simulink model "DLH_nguocslx"  (R2020a)
settings: Solver=VariableStepAuto  StartTime=0.0  StopTime=10.0  RelTol=1e-3
settings Model: Creator=dell  LastModifiedBy=dell

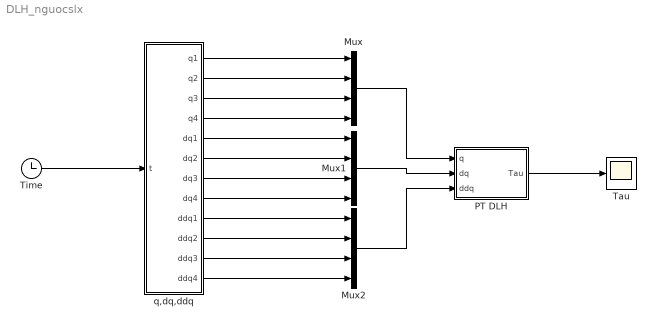
== system DLH_nguocslx ==
  Mux : Mux
  Mux1 : Mux
  Mux2 : Mux
  "PT DLH " : MATLAB Function  TreatAsAtomicUnit=on
  Tau : Scope
  Time : Clock
  q,dq,ddq : MATLAB Function  TreatAsAtomicUnit=on
  wires:
  Time/1 -> q,dq,ddq/1(t)
  q,dq,ddq/1(q1) -> Mux/1
  q,dq,ddq/2(q2) -> Mux/2
  q,dq,ddq/3(q3) -> Mux/3
  q,dq,ddq/4(q4) -> Mux/4
  q,dq,ddq/6(dq2) -> Mux1/2
  q,dq,ddq/5(dq1) -> Mux1/1
  q,dq,ddq/7(dq3) -> Mux1/3
  q,dq,ddq/8(dq4) -> Mux1/4
  q,dq,ddq/9(ddq1) -> Mux2/1
  q,dq,ddq/10(ddq2) -> Mux2/2
  q,dq,ddq/11(ddq3) -> Mux2/3
  q,dq,ddq/12(ddq4) -> Mux2/4
  Mux/1 -> "PT DLH "/1(q)
  Mux1/1 -> "PT DLH "/2(dq)
  Mux2/1 -> "PT DLH "/3(ddq)
  "PT DLH "/1(Tau) -> Tau/1

== matlab function DLH_nguocslx/PT DLH  ==
  data: q input; Tau output; dq input; ddq input
function Tau = fcn(q,dq,ddq)

[L1, L2, L3, L4,L0,m1,m2,m3,m4,I1x,I1y,I1z,I2x,I2y,I2z,I3x,I3y,I3z,I4x,I4y,I4z]=Parameters();

M=zeros(4,4);
M(1,1)= m1 + m2 + m3 + m4;
M(1,2)= ((-0.3e1 * m4 * L4 * cos(q(4)) - 0.3e1 * L3 * (m3 + 0.2e1 / 0.3e1 * m4)) * cos(q(3)) + 0.3e1 * sin(q(3)) * sin(q(4)) * L4 * m4 - 0.3e1 * L2 * (m2 + 0.2e1 / 0.3e1 * m3 + 0.2e1 / 0.3e1 * m4)) * cos(q(2)) / 0.2e1 + 0.3e1 / 0.2e1 * sin(q(2)) * (sin(q(4)) * L4 * m4 * cos(q(3)) + (m4 * L4 * cos(q(4)) + L3 * (m3 + 0.2e1 / 0.3e1 * m4)) * sin(q(3)));
M(1,3)= ((-0.3e1 * m4 * L4 * cos(q(4)) - 0.3e1 * L3 * (m3 + 0.2e1 / 0.3e1 * m4)) * cos(q(3)) + 0.3e1 * sin(q(3)) * sin(q(4)) * L4 * m4) * cos(q(2)) / 0.2e1 + 0.3e1 / 0.2e1 * sin(q(2)) * (sin(q(4)) * L4 * m4 * cos(q(3)) + (m4 * L4 * cos(q(4)) + L3 * (m3 + 0.2e1 / 0.3e1 * m4)) * sin(q(3)));
M(1,4)= 0.3e1 / 0.2e1 * L4 * ((sin(q(2)) * sin(q(3)) - cos(q(2)) * cos(q(3))) * cos(q(4)) + sin(q(4)) * (cos(q(2)) * sin(q(3)) + sin(q(2)) * cos(q(3)))) * m4;

M(2,1)= ((-0.3e1 * m4 * L4 * cos(q(4)) - 0.3e1 * L3 * (m3 + 0.2e1 / 0.3e1 * m4)) * cos(q(3)) + 0.3e1 * sin(q(3)) * sin(q(4)) * L4 * m4 - 0.3e1 * L2 * (m2 + 0.2e1 / 0.3e1 * m3 + 0.2e1 / 0.3e1 * m4)) * cos(q(2)) / 0.2e1 + 0.3e1 / 0.2e1 * sin(q(2)) * (sin(q(4)) * L4 * m4 * cos(q(3)) + (m4 * L4 * cos(q(4)) + L3 * (m3 + 0.2e1 / 0.3e1 * m4)) * sin(q(3)));
M(2,2)= 0.3e1 * L2 * (m4 * L4 * cos(q(4)) + L3 * (m3 + 0.2e1 / 0.3e1 * m4)) * cos(q(3)) + 0.3e1 * m4 * L4 * L3 * cos(q(4)) - 0.3e1 * m4 * L4 * L2 * sin(q(4)) * sin(q(3)) + ((9 * m2) + 0.4e1 * m3 + 0.4e1 * m4) * L2 ^ 2 / 0.4e1 + (0.4e1 * L3 ^ 2 + 0.9e1 * L4 ^ 2) * m4 / 0.4e1 + 0.9e1 / 0.4e1 * m3 * L3 ^ 2 + I3z + I4z + I2z;
M(2,3)= 0.3e1 / 0.2e1 * L2 * (m4 * L4 * cos(q(4)) + L3 * (m3 + 0.2e1 / 0.3e1 * m4)) * cos(q(3)) + 0.3e1 * m4 * L4 * L3 * cos(q(4)) - 0.3e1 / 0.2e1 * m4 * L4 * L2 * sin(q(4)) * sin(q(3)) + (0.4e1 * L3 ^ 2 + 0.9e1 * L4 ^ 2) * m4 / 0.4e1 + 0.9e1 / 0.4e1 * m3 * L3 ^ 2 + I3z + I4z;
M(2,4)= 0.3e1 / 0.2e1 * m4 * L4 * (L2 * cos(q(3)) + L3) * cos(q(4)) - 0.3e1 / 0.2e1 * m4 * L4 * L2 * sin(q(4)) * sin(q(3)) + 0.9e1 / 0.4e1 * m4 * L4 ^ 2 + I4z;

M(3,1)= ((-0.3e1 * m4 * L4 * cos(q(4)) - 0.3e1 * L3 * (m3 + 0.2e1 / 0.3e1 * m4)) * cos(q(3)) + 0.3e1 * sin(q(3)) * sin(q(4)) * L4 * m4) * cos(q(2)) / 0.2e1 + 0.3e1 / 0.2e1 * sin(q(2)) * (sin(q(4)) * L4 * m4 * cos(q(3)) + (m4 * L4 * cos(q(4)) + L3 * (m3 + 0.2e1 / 0.3e1 * m4)) * sin(q(3)));
M(3,2)= 0.3e1 / 0.2e1 * L2 * (m4 * L4 * cos(q(4)) + L3 * (m3 + 0.2e1 / 0.3e1 * m4)) * cos(q(3)) + 0.3e1 * m4 * L4 * L3 * cos(q(4)) - 0.3e1 / 0.2e1 * m4 * L4 * L2 * sin(q(4)) * sin(q(3)) + (0.4e1 * L3 ^ 2 + 0.9e1 * L4 ^ 2) * m4 / 0.4e1 + 0.9e1 / 0.4e1 * m3 * L3 ^ 2 + I3z + I4z;
M(3,3)= 0.3e1 * m4 * L4 * L3 * cos(q(4)) + ((9 * m3) + 0.4e1 * m4) * L3 ^ 2 / 0.4e1 + 0.9e1 / 0.4e1 * m4 * L4 ^ 2 + I3z + I4z;
M(3,4)= 0.3e1 / 0.2e1 * m4 * L4 * L3 * cos(q(4)) + 0.9e1 / 0.4e1 * m4 * L4 ^ 2 + I4z;

M(4,1)= 0.3e1 / 0.2e1 * L4 * ((sin(q(2)) * sin(q(3)) - cos(q(2)) * cos(q(3))) * cos(q(4)) + sin(q(4)) * (cos(q(2)) * sin(q(3)) + sin(q(2)) * cos(q(3)))) * m4;
M(4,2)= 0.3e1 / 0.2e1 * m4 * L4 * (L2 * cos(q(3)) + L3) * cos(q(4)) - 0.3e1 / 0.2e1 * m4 * L4 * L2 * sin(q(4)) * sin(q(3)) + 0.9e1 / 0.4e1 * m4 * L4 ^ 2 + I4z;
M(4,3)= 0.3e1 / 0.2e1 * m4 * L4 * L3 * cos(q(4)) + 0.9e1 / 0.4e1 * m4 * L4 ^ 2 + I4z;
M(4,4)= 0.9e1 / 0.4e1 * m4 * L4 ^ 2 + I4z;

C=zeros(4,4);

C(1,1)= 0;
C(1,2)= ((0.3e1 * L4 * m4 * (dq(3) + dq(4) + dq(2)) * cos(q(4)) + 0.3e1 * L3 * (dq(3) + dq(2)) * (m3 + 0.2e1 / 0.3e1 * m4)) * cos(q(3)) - 0.3e1 * sin(q(3)) * sin(q(4)) * L4 * m4 * (dq(3) + dq(4) + dq(2)) + 0.3e1 * dq(2) * L2 * (m2 + 0.2e1 / 0.3e1 * m3 + 0.2e1 / 0.3e1 * m4)) * sin(q(2)) / 0.2e1 + 0.3e1 / 0.2e1 * cos(q(2)) * (sin(q(4)) * L4 * m4 * (dq(3) + dq(4) + dq(2)) * cos(q(3)) + sin(q(3)) * (L4 * m4 * (dq(3) + dq(4) + dq(2)) * cos(q(4)) + L3 * (dq(3) + dq(2)) * (m3 + 0.2e1 / 0.3e1 * m4)));
C(1,3)= (0.3e1 * sin(q(4)) * L4 * m4 * (dq(3) + dq(4) + dq(2)) * cos(q(3)) + 0.3e1 * sin(q(3)) * (L4 * m4 * (dq(3) + dq(4) + dq(2)) * cos(q(4)) + L3 * (dq(3) + dq(2)) * (m3 + 0.2e1 / 0.3e1 * m4))) * cos(q(2)) / 0.2e1 + 0.3e1 / 0.2e1 * ((L4 * m4 * (dq(3) + dq(4) + dq(2)) * cos(q(4)) + L3 * (dq(3) + dq(2)) * (m3 + 0.2e1 / 0.3e1 * m4)) * cos(q(3)) - sin(q(3)) * sin(q(4)) * L4 * m4 * (dq(3) + dq(4) + dq(2))) * sin(q(2));
C(1,4)= 0.3e1 / 0.2e1 * L4 * ((cos(q(2)) * sin(q(3)) + sin(q(2)) * cos(q(3))) * cos(q(4)) + (cos(q(2)) * cos(q(3)) - sin(q(2)) * sin(q(3))) * sin(q(4))) * (dq(3) + dq(4) + dq(2)) * m4;

C(2,1)= ((0.3e1 * L4 * m4 * (dq(3) + dq(4) + dq(2)) * cos(q(4)) + 0.3e1 * L3 * (m3 + 0.2e1 / 0.3e1 * m4) * (dq(3) + dq(2))) * cos(q(3)) - 0.3e1 * sin(q(3)) * sin(q(4)) * L4 * m4 * (dq(3) + dq(4) + dq(2)) + 0.3e1 * dq(2) * L2 * (m2 + 0.2e1 / 0.3e1 * m3 + 0.2e1 / 0.3e1 * m4)) * sin(q(2)) / 0.4e1 + 0.3e1 / 0.4e1 * cos(q(2)) * (sin(q(4)) * L4 * m4 * (dq(3) + dq(4) + dq(2)) * cos(q(3)) + sin(q(3)) * (L4 * m4 * (dq(3) + dq(4) + dq(2)) * cos(q(4)) + L3 * (m3 + 0.2e1 / 0.3e1 * m4) * (dq(3) + dq(2))));
C(2,2)= (0.3e1 * sin(q(2)) * sin(q(4)) * L4 * m4 * dq(1) - 0.3e1 * (m4 * L4 * cos(q(4)) + L3 * (m3 + 0.2e1 / 0.3e1 * m4)) * dq(1) * cos(q(2)) - 0.12e2 * (L4 * m4 * (dq(4) + dq(3)) * cos(q(4)) + dq(3) * L3 * (m3 + 0.2e1 / 0.3e1 * m4)) * L2) * sin(q(3)) / 0.4e1 - 0.3e1 / 0.4e1 * dq(1) * ((m4 * L4 * cos(q(4)) + L3 * (m3 + 0.2e1 / 0.3e1 * m4)) * cos(q(3)) + L2 * (m2 + 0.2e1 / 0.3e1 * m3 + 0.2e1 / 0.3e1 * m4)) * sin(q(2)) - 0.3e1 * m4 * ((cos(q(2)) * dq(1) / 0.4e1 + L2 * (dq(4) + dq(3))) * cos(q(3)) + dq(4) * L3) * sin(q(4)) * L4;
C(2,3)= (0.3e1 * sin(q(2)) * sin(q(4)) * L4 * m4 * dq(1) - 0.3e1 * (m4 * L4 * cos(q(4)) + L3 * (m3 + 0.2e1 / 0.3e1 * m4)) * dq(1) * cos(q(2)) - 0.6e1 * (L4 * m4 * (dq(4) + dq(3)) * cos(q(4)) + dq(3) * L3 * (m3 + 0.2e1 / 0.3e1 * m4)) * L2) * sin(q(3)) / 0.4e1 + (-0.6e1 * L4 * m4 * (cos(q(2)) * dq(1) / 0.2e1 + L2 * (dq(4) + dq(3))) * sin(q(4)) - 0.3e1 * (m4 * L4 * cos(q(4)) + L3 * (m3 + 0.2e1 / 0.3e1 * m4)) * dq(1) * sin(q(2))) * cos(q(3)) / 0.4e1 - 0.3e1 * m4 * L4 * L3 * sin(q(4)) * dq(4);
C(2,4)= -0.3e1 / 0.2e1 * (((cos(q(2)) * dq(1) / 0.2e1 + L2 * (dq(4) + dq(3))) * cos(q(3)) - sin(q(2)) * sin(q(3)) * dq(1) / 0.2e1 + dq(4) * L3) * sin(q(4)) + (sin(q(2)) * dq(1) * cos(q(3)) / 0.2e1 + sin(q(3)) * (cos(q(2)) * dq(1) / 0.2e1 + L2 * (dq(4) + dq(3)))) * cos(q(4))) * L4 * m4;

C(3,1)= (0.3e1 * sin(q(4)) * L4 * m4 * (dq(3) + dq(4) + dq(2)) * cos(q(3)) + 0.3e1 * sin(q(3)) * (L4 * m4 * (dq(3) + dq(4) + dq(2)) * cos(q(4)) + L3 * (m3 + 0.2e1 / 0.3e1 * m4) * (dq(3) + dq(2)))) * cos(q(2)) / 0.4e1 + 0.3e1 / 0.4e1 * sin(q(2)) * ((L4 * m4 * (dq(3) + dq(4) + dq(2)) * cos(q(4)) + L3 * (m3 + 0.2e1 / 0.3e1 * m4) * (dq(3) + dq(2))) * cos(q(3)) - sin(q(3)) * sin(q(4)) * L4 * m4 * (dq(3) + dq(4) + dq(2)));
C(3,2)= (0.3e1 * sin(q(2)) * sin(q(4)) * L4 * m4 * dq(1) + 0.6e1 * L4 * m4 * (-cos(q(2)) * dq(1) / 0.2e1 + L2 * (dq(2) - dq(3) / 0.2e1 - dq(4) / 0.2e1)) * cos(q(4)) + 0.6e1 * (m3 + 0.2e1 / 0.3e1 * m4) * L3 * (-cos(q(2)) * dq(1) / 0.2e1 + L2 * (dq(2) - dq(3) / 0.2e1))) * sin(q(3)) / 0.4e1 + (0.6e1 * L4 * m4 * (-cos(q(2)) * dq(1) / 0.2e1 + L2 * (dq(2) - dq(3) / 0.2e1 - dq(4) / 0.2e1)) * sin(q(4)) - 0.3e1 * (m4 * L4 * cos(q(4)) + L3 * (m3 + 0.2e1 / 0.3e1 * m4)) * dq(1) * sin(q(2))) * cos(q(3)) / 0.4e1 - 0.3e1 * m4 * L4 * L3 * sin(q(4)) * dq(4);
C(3,3)= (-0.3e1 * (m4 * L4 * cos(q(4)) + L3 * (m3 + 0.2e1 / 0.3e1 * m4)) * dq(1) * cos(q(2)) + 0.3e1 * sin(q(2)) * sin(q(4)) * L4 * m4 * dq(1) + 0.3e1 * dq(2) * L2 * (m4 * L4 * cos(q(4)) + L3 * (m3 + 0.2e1 / 0.3e1 * m4))) * sin(q(3)) / 0.4e1 + (-0.3e1 * cos(q(2)) * sin(q(4)) * L4 * m4 * dq(1) - 0.3e1 * (m4 * L4 * cos(q(4)) + L3 * (m3 + 0.2e1 / 0.3e1 * m4)) * dq(1) * sin(q(2)) + 0.3e1 * L2 * dq(2) * sin(q(4)) * L4 * m4) * cos(q(3)) / 0.4e1 - 0.3e1 * m4 * L4 * L3 * sin(q(4)) * dq(4);
C(3,4)= 0.3e1 / 0.4e1 * (((L2 * dq(2) - cos(q(2)) * dq(1)) * cos(q(3)) + sin(q(2)) * sin(q(3)) * dq(1) - (2 * dq(4) * L3)) * sin(q(4)) + cos(q(4)) * (-sin(q(2)) * dq(1) * cos(q(3)) + sin(q(3)) * (L2 * dq(2) - cos(q(2)) * dq(1)))) * L4 * m4;

C(4,1)= 0.3e1 / 0.4e1 * L4 * (dq(3) + dq(4) + dq(2)) * m4 * ((cos(q(2)) * sin(q(3)) + sin(q(2)) * cos(q(3))) * cos(q(4)) + (cos(q(2)) * cos(q(3)) - sin(q(2)) * sin(q(3))) * sin(q(4)));
C(4,2)= -0.3e1 / 0.4e1 * L4 * m4 * (((cos(q(2)) * dq(1) + (L2 * (dq(3) + dq(4) - 2 * dq(2)))) * cos(q(3)) - sin(q(2)) * sin(q(3)) * dq(1) - 0.2e1 * (dq(3) - dq(4) / 0.2e1 + dq(2)) * L3) * sin(q(4)) + (sin(q(2)) * dq(1) * cos(q(3)) + (cos(q(2)) * dq(1) + (L2 * (dq(3) + dq(4) - 2 * dq(2)))) * sin(q(3))) * cos(q(4)));
C(4,3)= 0.3e1 / 0.4e1 * (((L2 * dq(2) - cos(q(2)) * dq(1)) * cos(q(3)) + sin(q(2)) * sin(q(3)) * dq(1) + 0.2e1 * (dq(3) - dq(4) / 0.2e1 + dq(2)) * L3) * sin(q(4)) + cos(q(4)) * (-sin(q(2)) * dq(1) * cos(q(3)) + sin(q(3)) * (L2 * dq(2) - cos(q(2)) * dq(1)))) * L4 * m4;
C(4,4)= 0.3e1 / 0.4e1 * L4 * (((L2 * dq(2) - cos(q(2)) * dq(1)) * cos(q(3)) + sin(q(2)) * sin(q(3)) * dq(1) + L3 * (dq(3) + dq(2))) * sin(q(4)) + cos(q(4)) * (-sin(q(2)) * dq(1) * cos(q(3)) + sin(q(3)) * (L2 * dq(2) - cos(q(2)) * dq(1)))) * m4;

G=zeros(4,1);
G(1,1)=0;
G(2,1)= -((15*m4*L4*cos(q(4)) + 15*L3*(m3 + (2*m4)/3))*cos(q(3)) - 15*sin(q(3))*sin(q(4))*L4*m4 + 15*L2*(m2 + (2*m3)/3 + (2*m4)/3))*sin(q(2)) - 15*m4*L4*cos(q(2))*sin(q(4))*cos(q(3)) - 15*sin(q(3))*(m4*L4*cos(q(4)) + L3*(m3 + (2*m4)/3))*cos(q(2));
G(3,1)= (-(15*m4*L4*cos(q(4)) + 15*L3*(m3 + (2*m4)/3))*sin(q(3)) - 15*sin(q(4))*L4*m4*cos(q(3)))*cos(q(2)) + 15*L4*sin(q(2))*sin(q(4))*sin(q(3))*m4 - 15*cos(q(3))*(m4*L4*cos(q(4)) + L3*(m3 + (2*m4)/3))*sin(q(2));
G(4,1)= (-15*sin(q(4))*L4*m4*cos(q(3)) - 15*sin(q(3))*cos(q(4))*L4*m4)*cos(q(2)) - 15*L4*sin(q(2))*cos(q(4))*cos(q(3))*m4 + 15*L4*sin(q(2))*sin(q(4))*sin(q(3))*m4;

Tau=M*ddq+C*dq+G;

== matlab function DLH_nguocslx/q,dq,ddq ==
  data: t input; q1 output; q2 output; q3 output; q4 output; dq1 output; dq2 output; dq3 output; dq4 output; ddq1 output; ddq2 output; ddq3 output; ddq4 output
function [q1,q2,q3,q4,dq1,dq2,dq3,dq4,ddq1,ddq2,ddq3,ddq4] = fcn(t)

q1=2*sin(t);
q2=2*cos(t);
q3=-2*sin(t);
q4=-2*cos(t);


dq1=2*cos(t);
dq2=-2*sin(t);
dq3=-2*cos(t);
dq4=2*sin(t);

ddq1=-2*sin(t);
ddq2=-2*cos(t);
ddq3=2*sin(t);
ddq4=2*cos(t);
